simulink model "load_test"  (R2015b)
settings: Solver=FixedStepDiscrete  StartTime=0.0  StopTime=inf  FixedStep=.001  RelTol=1e-3
PostLoadFcn:
  | build_location = fullfile(fileparts(which(bdroot)),'build');
  | set_param(0, 'CacheFolder', build_location);
  | set_param(0, 'CodeGenFolder', build_location);
InitFcn:
  | initialize
libraries: xpcethercatlib x10
settings Model: SimulationMode=external  Creator=rtheyyun  LastModifiedBy=Nick Tsutsunava
settings SolverCC: EnableConcurrentExecution=on  ConcurrentTasks=on
settings DataIOCC: SaveFinalState=on  SaveFormat=StructureWithTime  SignalLoggingSaveFormat=ModelDataLogs  InspectSignalLogs=on
settings OptimizationCC: BlockReduction=off  OptimizeBlockIOStorage=off  BufferReuse=off  GlobalBufferReuse=off  ExpressionFolding=off  ExpressionDepthLimit=2147483647  LocalBlockOutputs=off
settings DebuggingCC: ReadBeforeWriteMsg=DisableAll  WriteAfterWriteMsg=DisableAll  WriteAfterReadMsg=DisableAll  UnderspecifiedInitializationDetection=Classic  MergeDetectMultiDrivingBlocksExec=none  SolverPrmCheckMsg=warning  InheritedTsInSrcMsg=none  FcnCallInpInsideContextMsg=UseLocalSettings  StateNameClashWarn=warning
settings HardwareCC: ProdBitPerPointer=32  ProdLargestAtomicFloat=None  ProdWordSize=32  ProdLongLongMode=on  ProdHWDeviceType=Generic->32-bit x86 compatible
settings RTWCC: SystemTargetFile=slrt.tlc  TemplateMakefile=slrt_default_tmf  Description=Simulink Real-Time  RTWVerbose=off  RTWCompilerOptimization=on
settings SimulinkRealTimeCC: GeneratePreprocessorConditionals=Disable all  xPCisModelTimeout=off  xPCModelTimeoutSecs=20  xPCConcurrentTasks=on
settings ConfigComp: CovModelRefEnable=Off  CovSFcnEnable=off

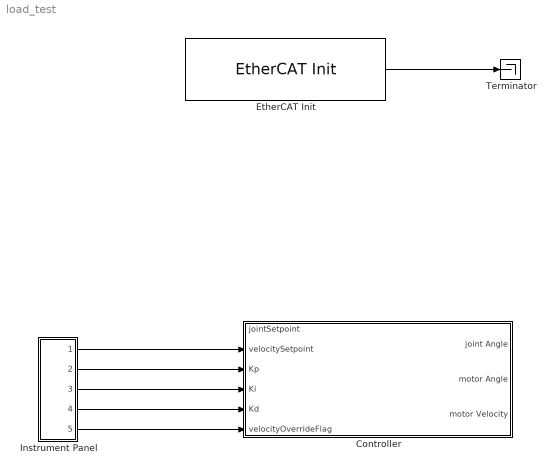
== system load_test ==
  Controller : Subsystem
  "EtherCAT Init " : xpcethercatlib/EtherCAT Init   Priority=0  config_file=C:\Users\rafae\Documents\GitHub\simulink-models\EtherCAT Config files\quad_slave_both_legs_v1.0.xml  device_id=0  pci_bus=2  pci_slot=0  dctuning=0  enaDebug=off  enaDC=on  errLink=off  masterDbg=off  stateChgDbg=off  baseClock=off  masterCfg=off  logFile='c:\dbglog.txt'  sample_time=0.001000
  Instrument Panel : Subsystem
  Terminator : Terminator
  wires:
  "EtherCAT Init "/1 -> Terminator/1
  Instrument Panel/1(Out2) -> Controller/2("velocitySetpoint ")
  Instrument Panel/2(Out3) -> Controller/3(Kp)
  Instrument Panel/3(Out4) -> Controller/4(Ki)
  Instrument Panel/4(Out5) -> Controller/5(Kd)
  Instrument Panel/5(Out6) -> Controller/6(velocityOverrideFlag)

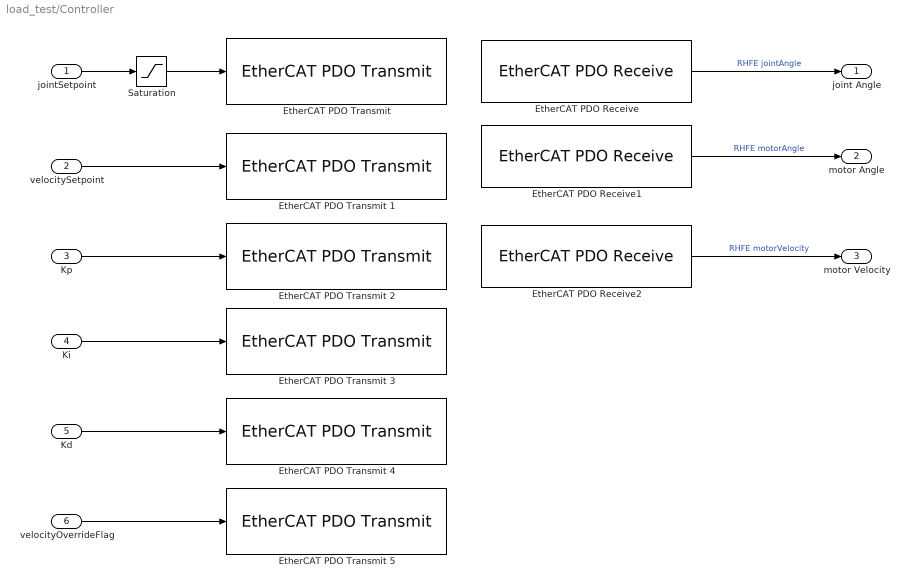
== system load_test/Controller ==
  jointSetpoint : Inport
  "velocitySetpoint " : Inport  Port=2
  Kp : Inport  Port=3
  Ki : Inport  Port=4
  Kd : Inport  Port=5
  velocityOverrideFlag : Inport  Port=6
  EtherCAT PDO Receive : xpcethercatlib/EtherCAT PDO Receive  Priority=2  sig_name=RHFE.Inputs.jointAngle  sig_offset=12496  sig_type=uint32  type_size=32  sig_dim=1  device_id=0  sample_time=0.001000
  EtherCAT PDO Receive1 : xpcethercatlib/EtherCAT PDO Receive  Priority=2  sig_name=RHFE.Inputs.motorAngle  sig_offset=12528  sig_type=uint16  type_size=16  sig_dim=1  device_id=0  sample_time=0.001000
  EtherCAT PDO Receive2 : xpcethercatlib/EtherCAT PDO Receive  Priority=2  sig_name=RHFE.Inputs.motorVelocity  sig_offset=12544  sig_type=int16  type_size=16  sig_dim=1  device_id=0  sample_time=0.001000
  "EtherCAT PDO Transmit " : xpcethercatlib/EtherCAT PDO Transmit   Priority=3  sig_name=RHFE.Outputs.jointSetpoint  sig_offset=12496  sig_type=uint32  type_size=32  sig_dim=1  device_id=0  sample_time=0.001000
  EtherCAT PDO Transmit 1 : xpcethercatlib/EtherCAT PDO Transmit   Priority=3  sig_name=RHFE.Outputs.data0  sig_offset=12528  sig_type=uint32  type_size=32  sig_dim=1  device_id=0  sample_time=0.001000
  EtherCAT PDO Transmit 2 : xpcethercatlib/EtherCAT PDO Transmit   Priority=3  sig_name=RHFE.Outputs.data1  sig_offset=12560  sig_type=uint32  type_size=32  sig_dim=1  device_id=0  sample_time=0.001000
  EtherCAT PDO Transmit 3 : xpcethercatlib/EtherCAT PDO Transmit   Priority=3  sig_name=RHFE.Outputs.data2  sig_offset=12592  sig_type=uint32  type_size=32  sig_dim=1  device_id=0  sample_time=0.001000
  EtherCAT PDO Transmit 4 : xpcethercatlib/EtherCAT PDO Transmit   Priority=3  sig_name=RHFE.Outputs.data3  sig_offset=12624  sig_type=uint32  type_size=32  sig_dim=1  device_id=0  sample_time=0.001000
  EtherCAT PDO Transmit 5 : xpcethercatlib/EtherCAT PDO Transmit   Priority=3  sig_name=RHFE.Outputs.data4  sig_offset=12656  sig_type=uint32  type_size=32  sig_dim=1  device_id=0  sample_time=0.001000
  Saturation : Saturate  UpperLimit=435000  LowerLimit=342000
  joint Angle : Outport
  motor Angle : Outport  Port=2
  motor Velocity : Outport  Port=3
  wires:
  Ki/1 -> EtherCAT PDO Transmit 3/1
  Kd/1 -> EtherCAT PDO Transmit 4/1
  EtherCAT PDO Receive/1 -> joint Angle/1  "RHFE jointAngle"
  jointSetpoint/1 -> Saturation/1
  "velocitySetpoint "/1 -> EtherCAT PDO Transmit 1/1
  EtherCAT PDO Receive2/1 -> motor Velocity/1  "RHFE motorVelocity"
  EtherCAT PDO Receive1/1 -> motor Angle/1  "RHFE motorAngle"
  velocityOverrideFlag/1 -> EtherCAT PDO Transmit 5/1
  Kp/1 -> EtherCAT PDO Transmit 2/1
  Saturation/1 -> "EtherCAT PDO Transmit "/1

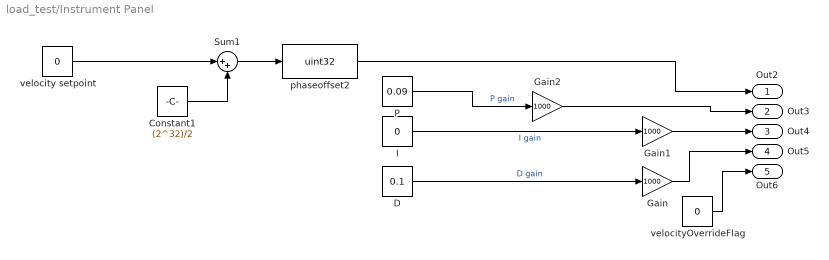
== system load_test/Instrument Panel ==
  Constant1 : Constant  Value=(2^32)/2
  D : Constant  Value=0.1  OutDataTypeStr=single
  Gain : Gain  Gain=1000  OutDataTypeStr=uint32
  Gain1 : Gain  Gain=1000  OutDataTypeStr=uint32
  Gain2 : Gain  Gain=1000  OutDataTypeStr=uint32
  I : Constant  Value=0  OutDataTypeStr=single
  P : Constant  Value=0.09  OutDataTypeStr=single
  Sum1 : Sum  Inputs=|++
  phaseoffset2 : DataTypeConversion  OutDataTypeStr=uint32
  velocity setpoint : Constant  Value=0  OutDataTypeStr=int16
  velocityOverrideFlag : Constant  Value=0  OutDataTypeStr=uint32
  Out2 : Outport
  Out3 : Outport  Port=2
  Out4 : Outport  Port=3
  Out5 : Outport  Port=4
  Out6 : Outport  Port=5
  wires:
  velocityOverrideFlag/1 -> Out6/1
  Gain2/1 -> Out3/1
  Constant1/1 -> Sum1/2
  Sum1/1 -> phaseoffset2/1
  velocity setpoint/1 -> Sum1/1
  phaseoffset2/1 -> Out2/1
  Gain1/1 -> Out4/1
  Gain/1 -> Out5/1
  I/1 -> Gain1/1  "I gain"
  D/1 -> Gain/1  "D gain"
  P/1 -> Gain2/1  "P gain"
